simulink model "PowerFlow_SUSAN"  (R2022b)
settings: Solver=FixedStepAuto  StartTime=0.0  StopTime=10  FixedStep=0.02  RelTol=1e-3
libraries: Lib_EMTAT x193
(part 2 of 3)

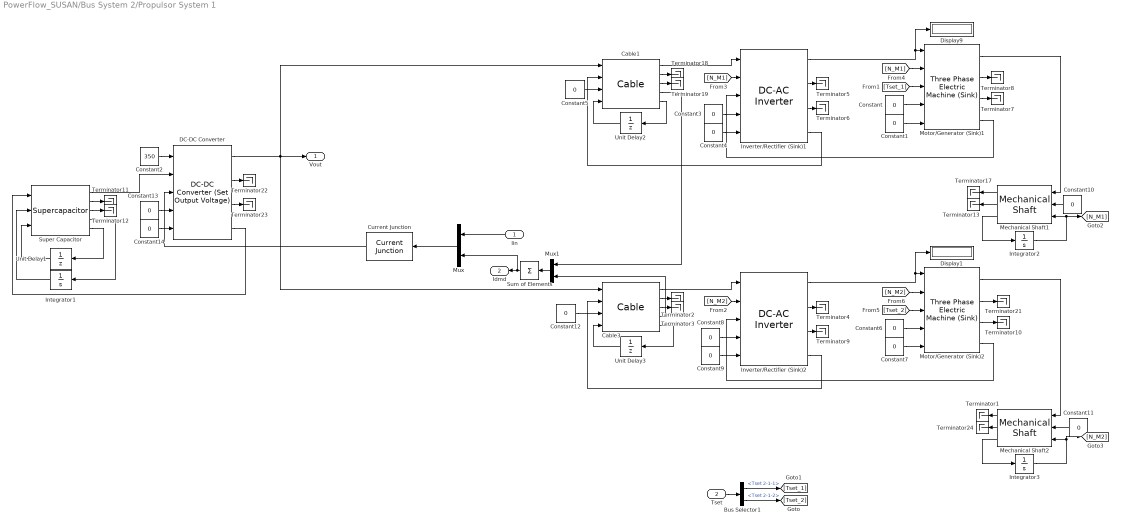
== system PowerFlow_SUSAN/Bus System 2/Propulsor System 1 ==
  Iin : Inport
  Tset : Inport  Port=2
  Bus Selector1 : BusSelector  OutputSignals=Tset 2-1-1,Tset 2-1-2
  Cable1 : Lib_EMTAT/Components/Power Flow/Cable  R=0.2
      settings: SourceProductName=EMTAT
  Cable3 : Lib_EMTAT/Components/Power Flow/Cable  R=0.2
      settings: SourceProductName=EMTAT
  Constant{,1,3..14} (14 alike) : Constant  Value=0
  Constant2 : Constant  Value=350
  Current Junction : Lib_EMTAT/Components/Power Flow/Current Junction  Nb=1
      settings: SourceProductName=EMTAT
      settings: AttributesFormatString=|
      | Current Junction
      | Version: %<LibraryVersion>
  DC-DC Converter : Lib_EMTAT/Components/Power Flow/DC-DC Converter (Set Output Voltage)  X_Vin_VoltageVec_M=[0 100 1000 5000]  Y_Iout_CurrentVec_M=[0 10 100 150]  T_C_PlossArray_M=0.98*ones(4,4)  FM=0  Plosslim=0
      settings: SourceProductName=EMTAT
  Display1 : Display
  Display9 : Display
  Integrator1 : Integrator  InitialCondition=150
  Integrator2 : Integrator  InitialCondition=2000
  Integrator3 : Integrator  InitialCondition=2000
  Inverter/Rectifier (Sink)1 : Lib_EMTAT/Components/Power Flow/DC-AC Inverter  X_C_VoltageInVec_M=[0 400]  Y_C_RMSCurrentOutVec_M=[0 300]  T_C_PowLossArray_M=[1000 1000;1000 1000]  K_e=0.0503  FM=0  Plosslim=0
      settings: SourceProductName=EMTAT
  Inverter/Rectifier (Sink)2 : Lib_EMTAT/Components/Power Flow/DC-AC Inverter  X_C_VoltageInVec_M=[0 400]  Y_C_RMSCurrentOutVec_M=[0 300]  T_C_PowLossArray_M=[1000 1000;1000 1000]  K_e=0.0503  FM=0  Plosslim=0
      settings: SourceProductName=EMTAT
  Mechanical Shaft1 : Lib_EMTAT/Components/Power Flow/Mechanical Shaft  J=0.01  B=0.001
      settings: SourceProductName=EMTAT
  Mechanical Shaft2 : Lib_EMTAT/Components/Power Flow/Mechanical Shaft  J=0.01  B=0.001
      settings: SourceProductName=EMTAT
  Motor/Generator (Sink)1 : Lib_EMTAT/Components/Power Flow/Three Phase Electric Machine (Sink)  X_C_SpeedVec_M=[0 100 1000 5000]  Y_C_TorqueVec_M=[0 10 100 150]  T_C_EffArray_M=0.99*ones(4,4)  FM=0
      settings: SourceProductName=EMTAT
  Motor/Generator (Sink)2 : Lib_EMTAT/Components/Power Flow/Three Phase Electric Machine (Sink)  X_C_SpeedVec_M=[0 100 1000 5000]  Y_C_TorqueVec_M=[0 10 100 150]  T_C_EffArray_M=0.99*ones(4,4)  FM=0
      settings: SourceProductName=EMTAT
  Mux : Mux  Inputs=2
  Mux1 : Mux  Inputs=2
  Sum of Elements : Sum  Inputs=+
  Super Capacitor : Lib_EMTAT/Components/Power Flow/Supercapacitor  C=130  ESR=0.02  TSE=0  BlkNm=double(gcb)
      settings: SourceProductName=EMTAT
  Terminator{1..13,17..19,21..24} (20 alike) : Terminator
  Unit Delay1 : UnitDelay  SampleTime=-1  HasFrameUpgradeWarning=on
  Unit Delay2 : UnitDelay  SampleTime=-1  HasFrameUpgradeWarning=on
  Unit Delay3 : UnitDelay  SampleTime=-1  HasFrameUpgradeWarning=on
  Vout : Outport
  Idmd : Outport  Port=2
  wires:
  Constant14/1 -> DC-DC Converter/5
  Constant13/1 -> DC-DC Converter/4
  Constant12/1 -> Cable3/3
  Mechanical Shaft2/2 -> Terminator24/1
  Mechanical Shaft2/1 -> Terminator1/1
  Constant11/1 -> Mechanical Shaft2/2
  Constant10/1 -> Mechanical Shaft1/2
  Mechanical Shaft1/3 -> Integrator2/1
  Motor/Generator (Sink)2/3 -> Terminator10/1
  Constant8/1 -> Inverter/Rectifier (Sink)2/4
  Inverter/Rectifier (Sink)2/1 -> Display1/1, Motor/Generator (Sink)2/1
  [N_M2] -> Motor/Generator (Sink)2/2
  Cable3/1 -> Inverter/Rectifier (Sink)2/1
  Motor/Generator (Sink)2/4 -> Inverter/Rectifier (Sink)2/3
  Constant6/1 -> Motor/Generator (Sink)2/4
  Inverter/Rectifier (Sink)2/4 -> Cable3/2
  [Tset_2] -> Motor/Generator (Sink)2/3
  Inverter/Rectifier (Sink)2/3 -> Terminator9/1
  [N_M2] -> Inverter/Rectifier (Sink)2/2
  Constant7/1 -> Motor/Generator (Sink)2/5
  Inverter/Rectifier (Sink)2/2 -> Terminator4/1
  Constant9/1 -> Inverter/Rectifier (Sink)2/5
  Constant5/1 -> Cable1/3
  Constant4/1 -> Inverter/Rectifier (Sink)1/5
  Constant3/1 -> Inverter/Rectifier (Sink)1/4
  Motor/Generator (Sink)1/3 -> Terminator7/1
  Constant1/1 -> Motor/Generator (Sink)1/5
  Constant/1 -> Motor/Generator (Sink)1/4
  Tset/1 -> Bus Selector1/1
  Bus Selector1/2 -> [Tset_2]  "<Tset 2-1-2>"
  Bus Selector1/1 -> [Tset_1]  "<Tset 2-1-1>"
  Sum of Elements/1 -> Idmd/1, Mux/2
  Mux1/1 -> Sum of Elements/1
  Motor/Generator (Sink)1/1 -> Mechanical Shaft1/1
  Inverter/Rectifier (Sink)1/2 -> Terminator5/1
  DC-DC Converter/3 -> Terminator23/1
  DC-DC Converter/2 -> Terminator22/1
  Mechanical Shaft1/1 -> Terminator17/1
  Motor/Generator (Sink)2/2 -> Terminator21/1
  Super Capacitor/3 -> Terminator12/1
  Cable1/2 -> Terminator18/1
  Motor/Generator (Sink)2/1 -> Mechanical Shaft2/1
  Cable3/3 -> Terminator3/1
  Motor/Generator (Sink)1/2 -> Terminator8/1
  Constant2/1 -> DC-DC Converter/1
  Cable1/4 -> Mux1/1
  Unit Delay1/1 -> Super Capacitor/3
  Super Capacitor/5 -> Unit Delay1/1
  Inverter/Rectifier (Sink)1/3 -> Terminator6/1
  Cable1/5 -> Unit Delay2/1
  Integrator1/1 -> Super Capacitor/2
  Inverter/Rectifier (Sink)1/4 -> Cable1/2
  Unit Delay3/1 -> Cable3/4
  Cable1/3 -> Terminator19/1
  Integrator3/1 -> Mechanical Shaft2/3, [N_M2]
  Cable3/4 -> Mux1/2
  Super Capacitor/2 -> Terminator11/1
  Inverter/Rectifier (Sink)1/1 -> Display9/1, Motor/Generator (Sink)1/1
  Cable3/5 -> Unit Delay3/1
  [N_M1] -> Inverter/Rectifier (Sink)1/2
  Cable1/1 -> Inverter/Rectifier (Sink)1/1
  Integrator2/1 -> Mechanical Shaft1/3, [N_M1]
  Mux/1 -> Current Junction/1
  Current Junction/1 -> DC-DC Converter/3
  DC-DC Converter/4 -> Super Capacitor/1
  Cable3/2 -> Terminator2/1
  Unit Delay2/1 -> Cable1/4
  Mechanical Shaft1/2 -> Terminator13/1
  [N_M1] -> Motor/Generator (Sink)1/2
  Super Capacitor/1 -> DC-DC Converter/2
  Super Capacitor/4 -> Integrator1/1
  Motor/Generator (Sink)1/4 -> Inverter/Rectifier (Sink)1/3
  DC-DC Converter/1 -> Cable1/1, Vout/1, Cable3/1
  [Tset_1] -> Motor/Generator (Sink)1/3
  Mechanical Shaft2/3 -> Integrator3/1
  Iin/1 -> Mux/1

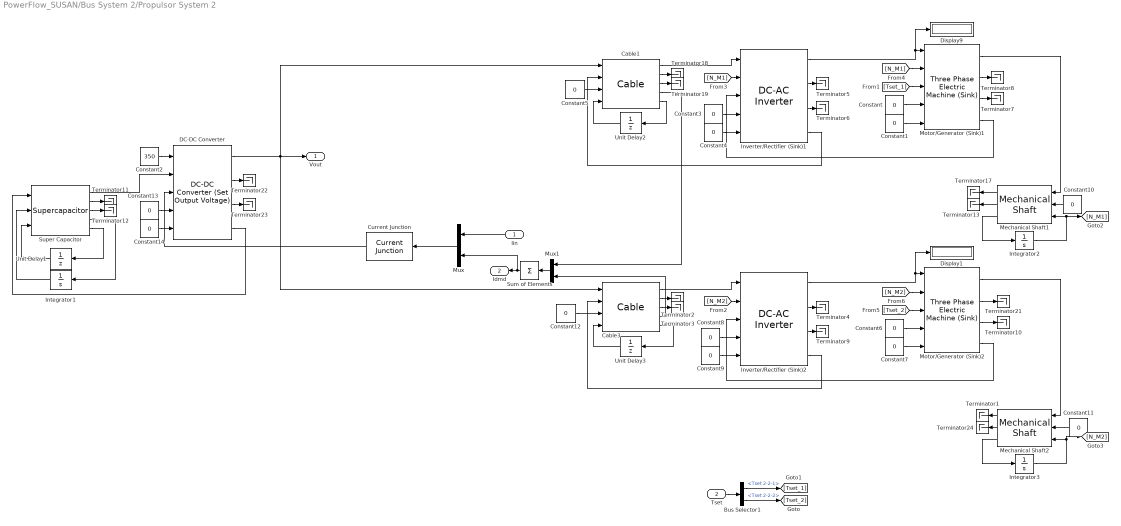
== system PowerFlow_SUSAN/Bus System 2/Propulsor System 2 ==
  Iin : Inport
  Tset : Inport  Port=2
  Bus Selector1 : BusSelector  OutputSignals=Tset 2-2-1,Tset 2-2-2
  Cable1 : Lib_EMTAT/Components/Power Flow/Cable  R=0.2
      settings: SourceProductName=EMTAT
  Cable3 : Lib_EMTAT/Components/Power Flow/Cable  R=0.2
      settings: SourceProductName=EMTAT
  Constant{,1,3..14} (14 alike) : Constant  Value=0
  Constant2 : Constant  Value=350
  Current Junction : Lib_EMTAT/Components/Power Flow/Current Junction  Nb=1
      settings: SourceProductName=EMTAT
      settings: AttributesFormatString=|
      | Current Junction
      | Version: %<LibraryVersion>
  DC-DC Converter : Lib_EMTAT/Components/Power Flow/DC-DC Converter (Set Output Voltage)  X_Vin_VoltageVec_M=[0 100 1000 5000]  Y_Iout_CurrentVec_M=[0 10 100 150]  T_C_PlossArray_M=0.98*ones(4,4)  FM=0  Plosslim=0
      settings: SourceProductName=EMTAT
  Display1 : Display
  Display9 : Display
  Integrator1 : Integrator  InitialCondition=150
  Integrator2 : Integrator  InitialCondition=2000
  Integrator3 : Integrator  InitialCondition=2000
  Inverter/Rectifier (Sink)1 : Lib_EMTAT/Components/Power Flow/DC-AC Inverter  X_C_VoltageInVec_M=[0 400]  Y_C_RMSCurrentOutVec_M=[0 300]  T_C_PowLossArray_M=[1000 1000;1000 1000]  K_e=0.0503  FM=0  Plosslim=0
      settings: SourceProductName=EMTAT
  Inverter/Rectifier (Sink)2 : Lib_EMTAT/Components/Power Flow/DC-AC Inverter  X_C_VoltageInVec_M=[0 400]  Y_C_RMSCurrentOutVec_M=[0 300]  T_C_PowLossArray_M=[1000 1000;1000 1000]  K_e=0.0503  FM=0  Plosslim=0
      settings: SourceProductName=EMTAT
  Mechanical Shaft1 : Lib_EMTAT/Components/Power Flow/Mechanical Shaft  J=0.01  B=0.001
      settings: SourceProductName=EMTAT
  Mechanical Shaft2 : Lib_EMTAT/Components/Power Flow/Mechanical Shaft  J=0.01  B=0.001
      settings: SourceProductName=EMTAT
  Motor/Generator (Sink)1 : Lib_EMTAT/Components/Power Flow/Three Phase Electric Machine (Sink)  X_C_SpeedVec_M=[0 100 1000 5000]  Y_C_TorqueVec_M=[0 10 100 150]  T_C_EffArray_M=0.99*ones(4,4)  FM=0
      settings: SourceProductName=EMTAT
  Motor/Generator (Sink)2 : Lib_EMTAT/Components/Power Flow/Three Phase Electric Machine (Sink)  X_C_SpeedVec_M=[0 100 1000 5000]  Y_C_TorqueVec_M=[0 10 100 150]  T_C_EffArray_M=0.99*ones(4,4)  FM=0
      settings: SourceProductName=EMTAT
  Mux : Mux  Inputs=2
  Mux1 : Mux  Inputs=2
  Sum of Elements : Sum  Inputs=+
  Super Capacitor : Lib_EMTAT/Components/Power Flow/Supercapacitor  C=130  ESR=0.02  TSE=0  BlkNm=double(gcb)
      settings: SourceProductName=EMTAT
  Terminator{1..13,17..19,21..24} (20 alike) : Terminator
  Unit Delay1 : UnitDelay  SampleTime=-1  HasFrameUpgradeWarning=on
  Unit Delay2 : UnitDelay  SampleTime=-1  HasFrameUpgradeWarning=on
  Unit Delay3 : UnitDelay  SampleTime=-1  HasFrameUpgradeWarning=on
  Vout : Outport
  Idmd : Outport  Port=2
  wires:
  Iin/1 -> Mux/1
  Mechanical Shaft2/3 -> Integrator3/1
  [Tset_1] -> Motor/Generator (Sink)1/3
  DC-DC Converter/1 -> Cable3/1, Vout/1, Cable1/1
  Motor/Generator (Sink)1/4 -> Inverter/Rectifier (Sink)1/3
  Super Capacitor/4 -> Integrator1/1
  Super Capacitor/1 -> DC-DC Converter/2
  [N_M1] -> Motor/Generator (Sink)1/2
  Mechanical Shaft1/2 -> Terminator13/1
  Unit Delay2/1 -> Cable1/4
  Cable3/2 -> Terminator2/1
  DC-DC Converter/4 -> Super Capacitor/1
  Current Junction/1 -> DC-DC Converter/3
  Mux/1 -> Current Junction/1
  Integrator2/1 -> [N_M1], Mechanical Shaft1/3
  Cable1/1 -> Inverter/Rectifier (Sink)1/1
  [N_M1] -> Inverter/Rectifier (Sink)1/2
  Cable3/5 -> Unit Delay3/1
  Inverter/Rectifier (Sink)1/1 -> Motor/Generator (Sink)1/1, Display9/1
  Super Capacitor/2 -> Terminator11/1
  Cable3/4 -> Mux1/2
  Integrator3/1 -> [N_M2], Mechanical Shaft2/3
  Cable1/3 -> Terminator19/1
  Unit Delay3/1 -> Cable3/4
  Inverter/Rectifier (Sink)1/4 -> Cable1/2
  Integrator1/1 -> Super Capacitor/2
  Cable1/5 -> Unit Delay2/1
  Inverter/Rectifier (Sink)1/3 -> Terminator6/1
  Super Capacitor/5 -> Unit Delay1/1
  Unit Delay1/1 -> Super Capacitor/3
  Cable1/4 -> Mux1/1
  Constant2/1 -> DC-DC Converter/1
  Motor/Generator (Sink)1/2 -> Terminator8/1
  Cable3/3 -> Terminator3/1
  Motor/Generator (Sink)2/1 -> Mechanical Shaft2/1
  Cable1/2 -> Terminator18/1
  Super Capacitor/3 -> Terminator12/1
  Motor/Generator (Sink)2/2 -> Terminator21/1
  Mechanical Shaft1/1 -> Terminator17/1
  DC-DC Converter/2 -> Terminator22/1
  DC-DC Converter/3 -> Terminator23/1
  Inverter/Rectifier (Sink)1/2 -> Terminator5/1
  Motor/Generator (Sink)1/1 -> Mechanical Shaft1/1
  Mux1/1 -> Sum of Elements/1
  Sum of Elements/1 -> Mux/2, Idmd/1
  Bus Selector1/1 -> [Tset_1]  "<Tset 2-2-1>"
  Bus Selector1/2 -> [Tset_2]  "<Tset 2-2-2>"
  Tset/1 -> Bus Selector1/1
  Constant/1 -> Motor/Generator (Sink)1/4
  Constant1/1 -> Motor/Generator (Sink)1/5
  Motor/Generator (Sink)1/3 -> Terminator7/1
  Constant3/1 -> Inverter/Rectifier (Sink)1/4
  Constant4/1 -> Inverter/Rectifier (Sink)1/5
  Constant5/1 -> Cable1/3
  Constant9/1 -> Inverter/Rectifier (Sink)2/5
  Inverter/Rectifier (Sink)2/2 -> Terminator4/1
  Constant7/1 -> Motor/Generator (Sink)2/5
  [N_M2] -> Inverter/Rectifier (Sink)2/2
  Inverter/Rectifier (Sink)2/3 -> Terminator9/1
  [Tset_2] -> Motor/Generator (Sink)2/3
  Inverter/Rectifier (Sink)2/4 -> Cable3/2
  Constant6/1 -> Motor/Generator (Sink)2/4
  Motor/Generator (Sink)2/4 -> Inverter/Rectifier (Sink)2/3
  Cable3/1 -> Inverter/Rectifier (Sink)2/1
  [N_M2] -> Motor/Generator (Sink)2/2
  Inverter/Rectifier (Sink)2/1 -> Motor/Generator (Sink)2/1, Display1/1
  Constant8/1 -> Inverter/Rectifier (Sink)2/4
  Motor/Generator (Sink)2/3 -> Terminator10/1
  Mechanical Shaft1/3 -> Integrator2/1
  Constant10/1 -> Mechanical Shaft1/2
  Constant11/1 -> Mechanical Shaft2/2
  Mechanical Shaft2/1 -> Terminator1/1
  Mechanical Shaft2/2 -> Terminator24/1
  Constant12/1 -> Cable3/3
  Constant13/1 -> DC-DC Converter/4
  Constant14/1 -> DC-DC Converter/5

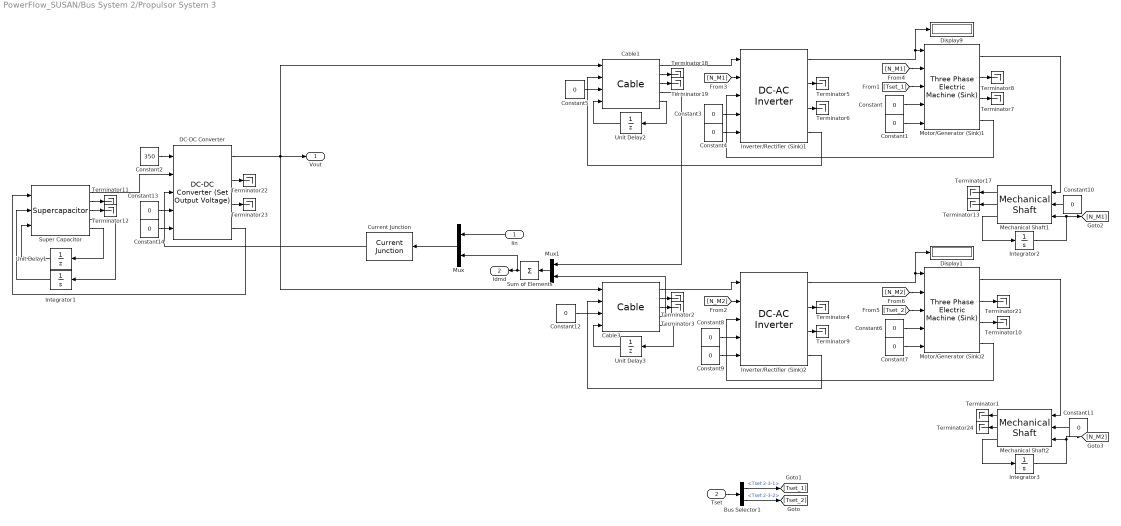
== system PowerFlow_SUSAN/Bus System 2/Propulsor System 3 ==
  Iin : Inport
  Tset : Inport  Port=2
  Bus Selector1 : BusSelector  OutputSignals=Tset 2-3-1,Tset 2-3-2
  Cable1 : Lib_EMTAT/Components/Power Flow/Cable  R=0.2
      settings: SourceProductName=EMTAT
  Cable3 : Lib_EMTAT/Components/Power Flow/Cable  R=0.2
      settings: SourceProductName=EMTAT
  Constant{,1,3..14} (14 alike) : Constant  Value=0
  Constant2 : Constant  Value=350
  Current Junction : Lib_EMTAT/Components/Power Flow/Current Junction  Nb=1
      settings: SourceProductName=EMTAT
      settings: AttributesFormatString=|
      | Current Junction
      | Version: %<LibraryVersion>
  DC-DC Converter : Lib_EMTAT/Components/Power Flow/DC-DC Converter (Set Output Voltage)  X_Vin_VoltageVec_M=[0 100 1000 5000]  Y_Iout_CurrentVec_M=[0 10 100 150]  T_C_PlossArray_M=0.98*ones(4,4)  FM=0  Plosslim=0
      settings: SourceProductName=EMTAT
  Display1 : Display
  Display9 : Display
  Integrator1 : Integrator  InitialCondition=150
  Integrator2 : Integrator  InitialCondition=2000
  Integrator3 : Integrator  InitialCondition=2000
  Inverter/Rectifier (Sink)1 : Lib_EMTAT/Components/Power Flow/DC-AC Inverter  X_C_VoltageInVec_M=[0 400]  Y_C_RMSCurrentOutVec_M=[0 300]  T_C_PowLossArray_M=[1000 1000;1000 1000]  K_e=0.0503  FM=0  Plosslim=0
      settings: SourceProductName=EMTAT
  Inverter/Rectifier (Sink)2 : Lib_EMTAT/Components/Power Flow/DC-AC Inverter  X_C_VoltageInVec_M=[0 400]  Y_C_RMSCurrentOutVec_M=[0 300]  T_C_PowLossArray_M=[1000 1000;1000 1000]  K_e=0.0503  FM=0  Plosslim=0
      settings: SourceProductName=EMTAT
  Mechanical Shaft1 : Lib_EMTAT/Components/Power Flow/Mechanical Shaft  J=0.01  B=0.001
      settings: SourceProductName=EMTAT
  Mechanical Shaft2 : Lib_EMTAT/Components/Power Flow/Mechanical Shaft  J=0.01  B=0.001
      settings: SourceProductName=EMTAT
  Motor/Generator (Sink)1 : Lib_EMTAT/Components/Power Flow/Three Phase Electric Machine (Sink)  X_C_SpeedVec_M=[0 100 1000 5000]  Y_C_TorqueVec_M=[0 10 100 150]  T_C_EffArray_M=0.99*ones(4,4)  FM=0
      settings: SourceProductName=EMTAT
  Motor/Generator (Sink)2 : Lib_EMTAT/Components/Power Flow/Three Phase Electric Machine (Sink)  X_C_SpeedVec_M=[0 100 1000 5000]  Y_C_TorqueVec_M=[0 10 100 150]  T_C_EffArray_M=0.99*ones(4,4)  FM=0
      settings: SourceProductName=EMTAT
  Mux : Mux  Inputs=2
  Mux1 : Mux  Inputs=2
  Sum of Elements : Sum  Inputs=+
  Super Capacitor : Lib_EMTAT/Components/Power Flow/Supercapacitor  C=130  ESR=0.02  TSE=0  BlkNm=double(gcb)
      settings: SourceProductName=EMTAT
  Terminator{1..13,17..19,21..24} (20 alike) : Terminator
  Unit Delay1 : UnitDelay  SampleTime=-1  HasFrameUpgradeWarning=on
  Unit Delay2 : UnitDelay  SampleTime=-1  HasFrameUpgradeWarning=on
  Unit Delay3 : UnitDelay  SampleTime=-1  HasFrameUpgradeWarning=on
  Vout : Outport
  Idmd : Outport  Port=2
  wires:
  Constant14/1 -> DC-DC Converter/5
  Constant13/1 -> DC-DC Converter/4
  Constant12/1 -> Cable3/3
  Mechanical Shaft2/2 -> Terminator24/1
  Mechanical Shaft2/1 -> Terminator1/1
  Constant11/1 -> Mechanical Shaft2/2
  Constant10/1 -> Mechanical Shaft1/2
  Mechanical Shaft1/3 -> Integrator2/1
  Motor/Generator (Sink)2/3 -> Terminator10/1
  Constant8/1 -> Inverter/Rectifier (Sink)2/4
  Inverter/Rectifier (Sink)2/1 -> Display1/1, Motor/Generator (Sink)2/1
  [N_M2] -> Motor/Generator (Sink)2/2
  Cable3/1 -> Inverter/Rectifier (Sink)2/1
  Motor/Generator (Sink)2/4 -> Inverter/Rectifier (Sink)2/3
  Constant6/1 -> Motor/Generator (Sink)2/4
  Inverter/Rectifier (Sink)2/4 -> Cable3/2
  [Tset_2] -> Motor/Generator (Sink)2/3
  Inverter/Rectifier (Sink)2/3 -> Terminator9/1
  [N_M2] -> Inverter/Rectifier (Sink)2/2
  Constant7/1 -> Motor/Generator (Sink)2/5
  Inverter/Rectifier (Sink)2/2 -> Terminator4/1
  Constant9/1 -> Inverter/Rectifier (Sink)2/5
  Constant5/1 -> Cable1/3
  Constant4/1 -> Inverter/Rectifier (Sink)1/5
  Constant3/1 -> Inverter/Rectifier (Sink)1/4
  Motor/Generator (Sink)1/3 -> Terminator7/1
  Constant1/1 -> Motor/Generator (Sink)1/5
  Constant/1 -> Motor/Generator (Sink)1/4
  Tset/1 -> Bus Selector1/1
  Bus Selector1/2 -> [Tset_2]  "<Tset 2-3-2>"
  Bus Selector1/1 -> [Tset_1]  "<Tset 2-3-1>"
  Sum of Elements/1 -> Idmd/1, Mux/2
  Mux1/1 -> Sum of Elements/1
  Motor/Generator (Sink)1/1 -> Mechanical Shaft1/1
  Inverter/Rectifier (Sink)1/2 -> Terminator5/1
  DC-DC Converter/3 -> Terminator23/1
  DC-DC Converter/2 -> Terminator22/1
  Mechanical Shaft1/1 -> Terminator17/1
  Motor/Generator (Sink)2/2 -> Terminator21/1
  Super Capacitor/3 -> Terminator12/1
  Cable1/2 -> Terminator18/1
  Motor/Generator (Sink)2/1 -> Mechanical Shaft2/1
  Cable3/3 -> Terminator3/1
  Motor/Generator (Sink)1/2 -> Terminator8/1
  Constant2/1 -> DC-DC Converter/1
  Cable1/4 -> Mux1/1
  Unit Delay1/1 -> Super Capacitor/3
  Super Capacitor/5 -> Unit Delay1/1
  Inverter/Rectifier (Sink)1/3 -> Terminator6/1
  Cable1/5 -> Unit Delay2/1
  Integrator1/1 -> Super Capacitor/2
  Inverter/Rectifier (Sink)1/4 -> Cable1/2
  Unit Delay3/1 -> Cable3/4
  Cable1/3 -> Terminator19/1
  Integrator3/1 -> Mechanical Shaft2/3, [N_M2]
  Cable3/4 -> Mux1/2
  Super Capacitor/2 -> Terminator11/1
  Inverter/Rectifier (Sink)1/1 -> Display9/1, Motor/Generator (Sink)1/1
  Cable3/5 -> Unit Delay3/1
  [N_M1] -> Inverter/Rectifier (Sink)1/2
  Cable1/1 -> Inverter/Rectifier (Sink)1/1
  Integrator2/1 -> Mechanical Shaft1/3, [N_M1]
  Mux/1 -> Current Junction/1
  Current Junction/1 -> DC-DC Converter/3
  DC-DC Converter/4 -> Super Capacitor/1
  Cable3/2 -> Terminator2/1
  Unit Delay2/1 -> Cable1/4
  Mechanical Shaft1/2 -> Terminator13/1
  [N_M1] -> Motor/Generator (Sink)1/2
  Super Capacitor/1 -> DC-DC Converter/2
  Super Capacitor/4 -> Integrator1/1
  Motor/Generator (Sink)1/4 -> Inverter/Rectifier (Sink)1/3
  DC-DC Converter/1 -> Cable1/1, Vout/1, Cable3/1
  [Tset_1] -> Motor/Generator (Sink)1/3
  Mechanical Shaft2/3 -> Integrator3/1
  Iin/1 -> Mux/1

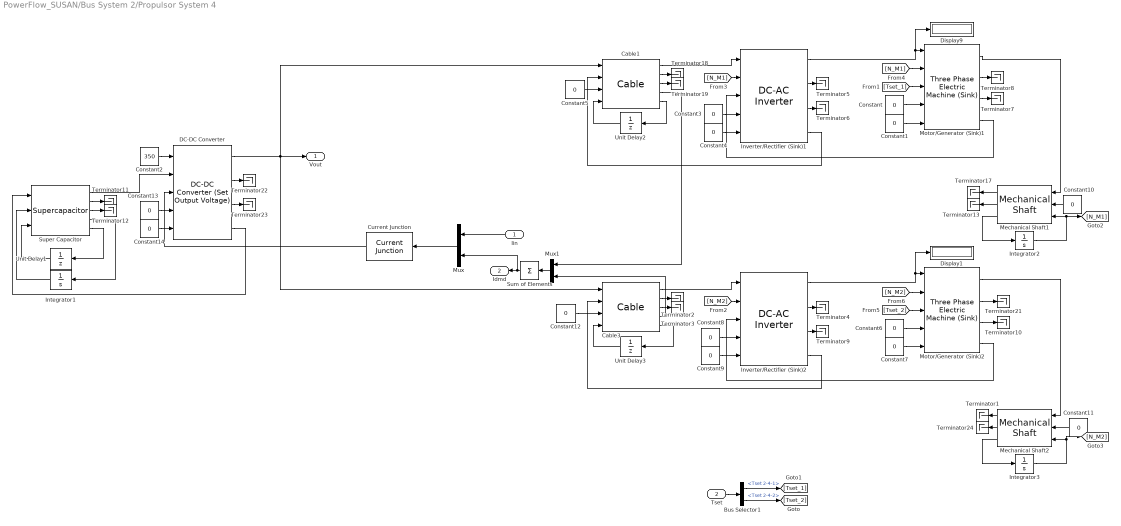
== system PowerFlow_SUSAN/Bus System 2/Propulsor System 4 ==
  Iin : Inport
  Tset : Inport  Port=2
  Bus Selector1 : BusSelector  OutputSignals=Tset 2-4-1,Tset 2-4-2
  Cable1 : Lib_EMTAT/Components/Power Flow/Cable  R=0.2
      settings: SourceProductName=EMTAT
  Cable3 : Lib_EMTAT/Components/Power Flow/Cable  R=0.2
      settings: SourceProductName=EMTAT
  Constant{,1,3..14} (14 alike) : Constant  Value=0
  Constant2 : Constant  Value=350
  Current Junction : Lib_EMTAT/Components/Power Flow/Current Junction  Nb=1
      settings: SourceProductName=EMTAT
      settings: AttributesFormatString=|
      | Current Junction
      | Version: %<LibraryVersion>
  DC-DC Converter : Lib_EMTAT/Components/Power Flow/DC-DC Converter (Set Output Voltage)  X_Vin_VoltageVec_M=[0 100 1000 5000]  Y_Iout_CurrentVec_M=[0 10 100 150]  T_C_PlossArray_M=0.98*ones(4,4)  FM=0  Plosslim=0
      settings: SourceProductName=EMTAT
  Display1 : Display
  Display9 : Display
  Integrator1 : Integrator  InitialCondition=150
  Integrator2 : Integrator  InitialCondition=2000
  Integrator3 : Integrator  InitialCondition=2000
  Inverter/Rectifier (Sink)1 : Lib_EMTAT/Components/Power Flow/DC-AC Inverter  X_C_VoltageInVec_M=[0 400]  Y_C_RMSCurrentOutVec_M=[0 300]  T_C_PowLossArray_M=[1000 1000;1000 1000]  K_e=0.0503  FM=0  Plosslim=0
      settings: SourceProductName=EMTAT
  Inverter/Rectifier (Sink)2 : Lib_EMTAT/Components/Power Flow/DC-AC Inverter  X_C_VoltageInVec_M=[0 400]  Y_C_RMSCurrentOutVec_M=[0 300]  T_C_PowLossArray_M=[1000 1000;1000 1000]  K_e=0.0503  FM=0  Plosslim=0
      settings: SourceProductName=EMTAT
  Mechanical Shaft1 : Lib_EMTAT/Components/Power Flow/Mechanical Shaft  J=0.01  B=0.001
      settings: SourceProductName=EMTAT
  Mechanical Shaft2 : Lib_EMTAT/Components/Power Flow/Mechanical Shaft  J=0.01  B=0.001
      settings: SourceProductName=EMTAT
  Motor/Generator (Sink)1 : Lib_EMTAT/Components/Power Flow/Three Phase Electric Machine (Sink)  X_C_SpeedVec_M=[0 100 1000 5000]  Y_C_TorqueVec_M=[0 10 100 150]  T_C_EffArray_M=0.99*ones(4,4)  FM=0
      settings: SourceProductName=EMTAT
  Motor/Generator (Sink)2 : Lib_EMTAT/Components/Power Flow/Three Phase Electric Machine (Sink)  X_C_SpeedVec_M=[0 100 1000 5000]  Y_C_TorqueVec_M=[0 10 100 150]  T_C_EffArray_M=0.99*ones(4,4)  FM=0
      settings: SourceProductName=EMTAT
  Mux : Mux  Inputs=2
  Mux1 : Mux  Inputs=2
  Sum of Elements : Sum  Inputs=+
  Super Capacitor : Lib_EMTAT/Components/Power Flow/Supercapacitor  C=130  ESR=0.02  TSE=0  BlkNm=double(gcb)
      settings: SourceProductName=EMTAT
  Terminator{1..13,17..19,21..24} (20 alike) : Terminator
  Unit Delay1 : UnitDelay  SampleTime=-1  HasFrameUpgradeWarning=on
  Unit Delay2 : UnitDelay  SampleTime=-1  HasFrameUpgradeWarning=on
  Unit Delay3 : UnitDelay  SampleTime=-1  HasFrameUpgradeWarning=on
  Vout : Outport
  Idmd : Outport  Port=2
  wires:
  Iin/1 -> Mux/1
  Mechanical Shaft2/3 -> Integrator3/1
  [Tset_1] -> Motor/Generator (Sink)1/3
  DC-DC Converter/1 -> Cable3/1, Vout/1, Cable1/1
  Motor/Generator (Sink)1/4 -> Inverter/Rectifier (Sink)1/3
  Super Capacitor/4 -> Integrator1/1
  Super Capacitor/1 -> DC-DC Converter/2
  [N_M1] -> Motor/Generator (Sink)1/2
  Mechanical Shaft1/2 -> Terminator13/1
  Unit Delay2/1 -> Cable1/4
  Cable3/2 -> Terminator2/1
  DC-DC Converter/4 -> Super Capacitor/1
  Current Junction/1 -> DC-DC Converter/3
  Mux/1 -> Current Junction/1
  Integrator2/1 -> [N_M1], Mechanical Shaft1/3
  Cable1/1 -> Inverter/Rectifier (Sink)1/1
  [N_M1] -> Inverter/Rectifier (Sink)1/2
  Cable3/5 -> Unit Delay3/1
  Inverter/Rectifier (Sink)1/1 -> Motor/Generator (Sink)1/1, Display9/1
  Super Capacitor/2 -> Terminator11/1
  Cable3/4 -> Mux1/2
  Integrator3/1 -> [N_M2], Mechanical Shaft2/3
  Cable1/3 -> Terminator19/1
  Unit Delay3/1 -> Cable3/4
  Inverter/Rectifier (Sink)1/4 -> Cable1/2
  Integrator1/1 -> Super Capacitor/2
  Cable1/5 -> Unit Delay2/1
  Inverter/Rectifier (Sink)1/3 -> Terminator6/1
  Super Capacitor/5 -> Unit Delay1/1
  Unit Delay1/1 -> Super Capacitor/3
  Cable1/4 -> Mux1/1
  Constant2/1 -> DC-DC Converter/1
  Motor/Generator (Sink)1/2 -> Terminator8/1
  Cable3/3 -> Terminator3/1
  Motor/Generator (Sink)2/1 -> Mechanical Shaft2/1
  Cable1/2 -> Terminator18/1
  Super Capacitor/3 -> Terminator12/1
  Motor/Generator (Sink)2/2 -> Terminator21/1
  Mechanical Shaft1/1 -> Terminator17/1
  DC-DC Converter/2 -> Terminator22/1
  DC-DC Converter/3 -> Terminator23/1
  Inverter/Rectifier (Sink)1/2 -> Terminator5/1
  Motor/Generator (Sink)1/1 -> Mechanical Shaft1/1
  Mux1/1 -> Sum of Elements/1
  Sum of Elements/1 -> Mux/2, Idmd/1
  Bus Selector1/1 -> [Tset_1]  "<Tset 2-4-1>"
  Bus Selector1/2 -> [Tset_2]  "<Tset 2-4-2>"
  Tset/1 -> Bus Selector1/1
  Constant/1 -> Motor/Generator (Sink)1/4
  Constant1/1 -> Motor/Generator (Sink)1/5
  Motor/Generator (Sink)1/3 -> Terminator7/1
  Constant3/1 -> Inverter/Rectifier (Sink)1/4
  Constant4/1 -> Inverter/Rectifier (Sink)1/5
  Constant5/1 -> Cable1/3
  Constant9/1 -> Inverter/Rectifier (Sink)2/5
  Inverter/Rectifier (Sink)2/2 -> Terminator4/1
  Constant7/1 -> Motor/Generator (Sink)2/5
  [N_M2] -> Inverter/Rectifier (Sink)2/2
  Inverter/Rectifier (Sink)2/3 -> Terminator9/1
  [Tset_2] -> Motor/Generator (Sink)2/3
  Inverter/Rectifier (Sink)2/4 -> Cable3/2
  Constant6/1 -> Motor/Generator (Sink)2/4
  Motor/Generator (Sink)2/4 -> Inverter/Rectifier (Sink)2/3
  Cable3/1 -> Inverter/Rectifier (Sink)2/1
  [N_M2] -> Motor/Generator (Sink)2/2
  Inverter/Rectifier (Sink)2/1 -> Motor/Generator (Sink)2/1, Display1/1
  Constant8/1 -> Inverter/Rectifier (Sink)2/4
  Motor/Generator (Sink)2/3 -> Terminator10/1
  Mechanical Shaft1/3 -> Integrator2/1
  Constant10/1 -> Mechanical Shaft1/2
  Constant11/1 -> Mechanical Shaft2/2
  Mechanical Shaft2/1 -> Terminator1/1
  Mechanical Shaft2/2 -> Terminator24/1
  Constant12/1 -> Cable3/3
  Constant13/1 -> DC-DC Converter/4
  Constant14/1 -> DC-DC Converter/5

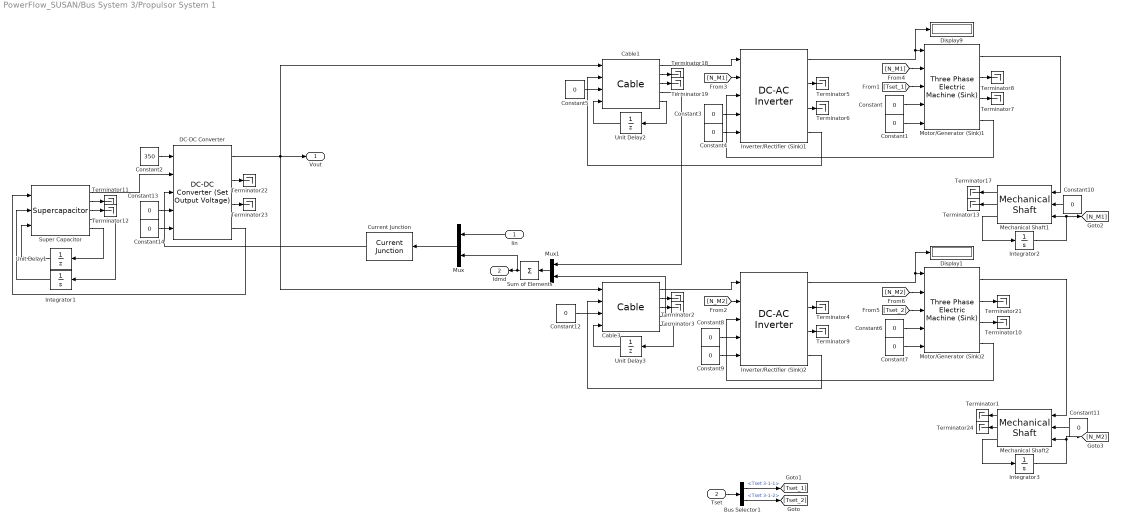
== system PowerFlow_SUSAN/Bus System 3/Propulsor System 1 ==
  Iin : Inport
  Tset : Inport  Port=2
  Bus Selector1 : BusSelector  OutputSignals=Tset 3-1-1,Tset 3-1-2
  Cable1 : Lib_EMTAT/Components/Power Flow/Cable  R=0.2
      settings: SourceProductName=EMTAT
  Cable3 : Lib_EMTAT/Components/Power Flow/Cable  R=0.2
      settings: SourceProductName=EMTAT
  Constant{,1,3..14} (14 alike) : Constant  Value=0
  Constant2 : Constant  Value=350
  Current Junction : Lib_EMTAT/Components/Power Flow/Current Junction  Nb=1
      settings: SourceProductName=EMTAT
      settings: AttributesFormatString=|
      | Current Junction
      | Version: %<LibraryVersion>
  DC-DC Converter : Lib_EMTAT/Components/Power Flow/DC-DC Converter (Set Output Voltage)  X_Vin_VoltageVec_M=[0 100 1000 5000]  Y_Iout_CurrentVec_M=[0 10 100 150]  T_C_PlossArray_M=0.98*ones(4,4)  FM=0  Plosslim=0
      settings: SourceProductName=EMTAT
  Display1 : Display
  Display9 : Display
  Integrator1 : Integrator  InitialCondition=150
  Integrator2 : Integrator  InitialCondition=2000
  Integrator3 : Integrator  InitialCondition=2000
  Inverter/Rectifier (Sink)1 : Lib_EMTAT/Components/Power Flow/DC-AC Inverter  X_C_VoltageInVec_M=[0 400]  Y_C_RMSCurrentOutVec_M=[0 300]  T_C_PowLossArray_M=[1000 1000;1000 1000]  K_e=0.0503  FM=0  Plosslim=0
      settings: SourceProductName=EMTAT
  Inverter/Rectifier (Sink)2 : Lib_EMTAT/Components/Power Flow/DC-AC Inverter  X_C_VoltageInVec_M=[0 400]  Y_C_RMSCurrentOutVec_M=[0 300]  T_C_PowLossArray_M=[1000 1000;1000 1000]  K_e=0.0503  FM=0  Plosslim=0
      settings: SourceProductName=EMTAT
  Mechanical Shaft1 : Lib_EMTAT/Components/Power Flow/Mechanical Shaft  J=0.01  B=0.001
      settings: SourceProductName=EMTAT
  Mechanical Shaft2 : Lib_EMTAT/Components/Power Flow/Mechanical Shaft  J=0.01  B=0.001
      settings: SourceProductName=EMTAT
  Motor/Generator (Sink)1 : Lib_EMTAT/Components/Power Flow/Three Phase Electric Machine (Sink)  X_C_SpeedVec_M=[0 100 1000 5000]  Y_C_TorqueVec_M=[0 10 100 150]  T_C_EffArray_M=0.99*ones(4,4)  FM=0
      settings: SourceProductName=EMTAT
  Motor/Generator (Sink)2 : Lib_EMTAT/Components/Power Flow/Three Phase Electric Machine (Sink)  X_C_SpeedVec_M=[0 100 1000 5000]  Y_C_TorqueVec_M=[0 10 100 150]  T_C_EffArray_M=0.99*ones(4,4)  FM=0
      settings: SourceProductName=EMTAT
  Mux : Mux  Inputs=2
  Mux1 : Mux  Inputs=2
  Sum of Elements : Sum  Inputs=+
  Super Capacitor : Lib_EMTAT/Components/Power Flow/Supercapacitor  C=130  ESR=0.02  TSE=0  BlkNm=double(gcb)
      settings: SourceProductName=EMTAT
  Terminator{1..13,17..19,21..24} (20 alike) : Terminator
  Unit Delay1 : UnitDelay  SampleTime=-1  HasFrameUpgradeWarning=on
  Unit Delay2 : UnitDelay  SampleTime=-1  HasFrameUpgradeWarning=on
  Unit Delay3 : UnitDelay  SampleTime=-1  HasFrameUpgradeWarning=on
  Vout : Outport
  Idmd : Outport  Port=2
  wires:
  Iin/1 -> Mux/1
  Mechanical Shaft2/3 -> Integrator3/1
  [Tset_1] -> Motor/Generator (Sink)1/3
  DC-DC Converter/1 -> Cable3/1, Vout/1, Cable1/1
  Motor/Generator (Sink)1/4 -> Inverter/Rectifier (Sink)1/3
  Super Capacitor/4 -> Integrator1/1
  Super Capacitor/1 -> DC-DC Converter/2
  [N_M1] -> Motor/Generator (Sink)1/2
  Mechanical Shaft1/2 -> Terminator13/1
  Unit Delay2/1 -> Cable1/4
  Cable3/2 -> Terminator2/1
  DC-DC Converter/4 -> Super Capacitor/1
  Current Junction/1 -> DC-DC Converter/3
  Mux/1 -> Current Junction/1
  Integrator2/1 -> [N_M1], Mechanical Shaft1/3
  Cable1/1 -> Inverter/Rectifier (Sink)1/1
  [N_M1] -> Inverter/Rectifier (Sink)1/2
  Cable3/5 -> Unit Delay3/1
  Inverter/Rectifier (Sink)1/1 -> Motor/Generator (Sink)1/1, Display9/1
  Super Capacitor/2 -> Terminator11/1
  Cable3/4 -> Mux1/2
  Integrator3/1 -> [N_M2], Mechanical Shaft2/3
  Cable1/3 -> Terminator19/1
  Unit Delay3/1 -> Cable3/4
  Inverter/Rectifier (Sink)1/4 -> Cable1/2
  Integrator1/1 -> Super Capacitor/2
  Cable1/5 -> Unit Delay2/1
  Inverter/Rectifier (Sink)1/3 -> Terminator6/1
  Super Capacitor/5 -> Unit Delay1/1
  Unit Delay1/1 -> Super Capacitor/3
  Cable1/4 -> Mux1/1
  Constant2/1 -> DC-DC Converter/1
  Motor/Generator (Sink)1/2 -> Terminator8/1
  Cable3/3 -> Terminator3/1
  Motor/Generator (Sink)2/1 -> Mechanical Shaft2/1
  Cable1/2 -> Terminator18/1
  Super Capacitor/3 -> Terminator12/1
  Motor/Generator (Sink)2/2 -> Terminator21/1
  Mechanical Shaft1/1 -> Terminator17/1
  DC-DC Converter/2 -> Terminator22/1
  DC-DC Converter/3 -> Terminator23/1
  Inverter/Rectifier (Sink)1/2 -> Terminator5/1
  Motor/Generator (Sink)1/1 -> Mechanical Shaft1/1
  Mux1/1 -> Sum of Elements/1
  Sum of Elements/1 -> Mux/2, Idmd/1
  Bus Selector1/1 -> [Tset_1]  "<Tset 3-1-1>"
  Bus Selector1/2 -> [Tset_2]  "<Tset 3-1-2>"
  Tset/1 -> Bus Selector1/1
  Constant/1 -> Motor/Generator (Sink)1/4
  Constant1/1 -> Motor/Generator (Sink)1/5
  Motor/Generator (Sink)1/3 -> Terminator7/1
  Constant3/1 -> Inverter/Rectifier (Sink)1/4
  Constant4/1 -> Inverter/Rectifier (Sink)1/5
  Constant5/1 -> Cable1/3
  Constant9/1 -> Inverter/Rectifier (Sink)2/5
  Inverter/Rectifier (Sink)2/2 -> Terminator4/1
  Constant7/1 -> Motor/Generator (Sink)2/5
  [N_M2] -> Inverter/Rectifier (Sink)2/2
  Inverter/Rectifier (Sink)2/3 -> Terminator9/1
  [Tset_2] -> Motor/Generator (Sink)2/3
  Inverter/Rectifier (Sink)2/4 -> Cable3/2
  Constant6/1 -> Motor/Generator (Sink)2/4
  Motor/Generator (Sink)2/4 -> Inverter/Rectifier (Sink)2/3
  Cable3/1 -> Inverter/Rectifier (Sink)2/1
  [N_M2] -> Motor/Generator (Sink)2/2
  Inverter/Rectifier (Sink)2/1 -> Motor/Generator (Sink)2/1, Display1/1
  Constant8/1 -> Inverter/Rectifier (Sink)2/4
  Motor/Generator (Sink)2/3 -> Terminator10/1
  Mechanical Shaft1/3 -> Integrator2/1
  Constant10/1 -> Mechanical Shaft1/2
  Constant11/1 -> Mechanical Shaft2/2
  Mechanical Shaft2/1 -> Terminator1/1
  Mechanical Shaft2/2 -> Terminator24/1
  Constant12/1 -> Cable3/3
  Constant13/1 -> DC-DC Converter/4
  Constant14/1 -> DC-DC Converter/5

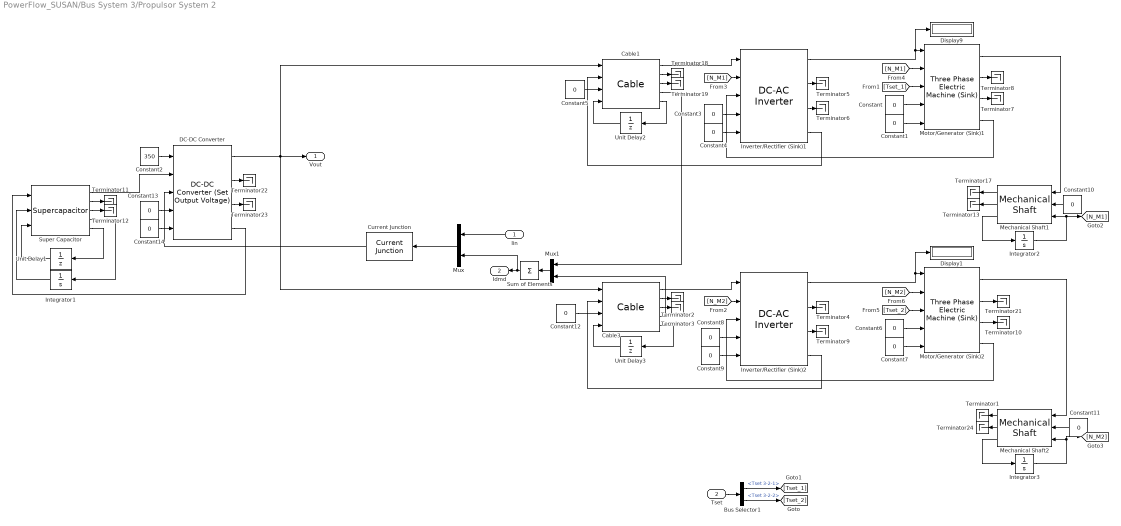
== system PowerFlow_SUSAN/Bus System 3/Propulsor System 2 ==
  Iin : Inport
  Tset : Inport  Port=2
  Bus Selector1 : BusSelector  OutputSignals=Tset 3-2-1,Tset 3-2-2
  Cable1 : Lib_EMTAT/Components/Power Flow/Cable  R=0.2
      settings: SourceProductName=EMTAT
  Cable3 : Lib_EMTAT/Components/Power Flow/Cable  R=0.2
      settings: SourceProductName=EMTAT
  Constant{,1,3..14} (14 alike) : Constant  Value=0
  Constant2 : Constant  Value=350
  Current Junction : Lib_EMTAT/Components/Power Flow/Current Junction  Nb=1
      settings: SourceProductName=EMTAT
      settings: AttributesFormatString=|
      | Current Junction
      | Version: %<LibraryVersion>
  DC-DC Converter : Lib_EMTAT/Components/Power Flow/DC-DC Converter (Set Output Voltage)  X_Vin_VoltageVec_M=[0 100 1000 5000]  Y_Iout_CurrentVec_M=[0 10 100 150]  T_C_PlossArray_M=0.98*ones(4,4)  FM=0  Plosslim=0
      settings: SourceProductName=EMTAT
  Display1 : Display
  Display9 : Display
  Integrator1 : Integrator  InitialCondition=150
  Integrator2 : Integrator  InitialCondition=2000
  Integrator3 : Integrator  InitialCondition=2000
  Inverter/Rectifier (Sink)1 : Lib_EMTAT/Components/Power Flow/DC-AC Inverter  X_C_VoltageInVec_M=[0 400]  Y_C_RMSCurrentOutVec_M=[0 300]  T_C_PowLossArray_M=[1000 1000;1000 1000]  K_e=0.0503  FM=0  Plosslim=0
      settings: SourceProductName=EMTAT
  Inverter/Rectifier (Sink)2 : Lib_EMTAT/Components/Power Flow/DC-AC Inverter  X_C_VoltageInVec_M=[0 400]  Y_C_RMSCurrentOutVec_M=[0 300]  T_C_PowLossArray_M=[1000 1000;1000 1000]  K_e=0.0503  FM=0  Plosslim=0
      settings: SourceProductName=EMTAT
  Mechanical Shaft1 : Lib_EMTAT/Components/Power Flow/Mechanical Shaft  J=0.01  B=0.001
      settings: SourceProductName=EMTAT
  Mechanical Shaft2 : Lib_EMTAT/Components/Power Flow/Mechanical Shaft  J=0.01  B=0.001
      settings: SourceProductName=EMTAT
  Motor/Generator (Sink)1 : Lib_EMTAT/Components/Power Flow/Three Phase Electric Machine (Sink)  X_C_SpeedVec_M=[0 100 1000 5000]  Y_C_TorqueVec_M=[0 10 100 150]  T_C_EffArray_M=0.99*ones(4,4)  FM=0
      settings: SourceProductName=EMTAT
  Motor/Generator (Sink)2 : Lib_EMTAT/Components/Power Flow/Three Phase Electric Machine (Sink)  X_C_SpeedVec_M=[0 100 1000 5000]  Y_C_TorqueVec_M=[0 10 100 150]  T_C_EffArray_M=0.99*ones(4,4)  FM=0
      settings: SourceProductName=EMTAT
  Mux : Mux  Inputs=2
  Mux1 : Mux  Inputs=2
  Sum of Elements : Sum  Inputs=+
  Super Capacitor : Lib_EMTAT/Components/Power Flow/Supercapacitor  C=130  ESR=0.02  TSE=0  BlkNm=double(gcb)
      settings: SourceProductName=EMTAT
  Terminator{1..13,17..19,21..24} (20 alike) : Terminator
  Unit Delay1 : UnitDelay  SampleTime=-1  HasFrameUpgradeWarning=on
  Unit Delay2 : UnitDelay  SampleTime=-1  HasFrameUpgradeWarning=on
  Unit Delay3 : UnitDelay  SampleTime=-1  HasFrameUpgradeWarning=on
  Vout : Outport
  Idmd : Outport  Port=2
  wires:
  Constant14/1 -> DC-DC Converter/5
  Constant13/1 -> DC-DC Converter/4
  Constant12/1 -> Cable3/3
  Mechanical Shaft2/2 -> Terminator24/1
  Mechanical Shaft2/1 -> Terminator1/1
  Constant11/1 -> Mechanical Shaft2/2
  Constant10/1 -> Mechanical Shaft1/2
  Mechanical Shaft1/3 -> Integrator2/1
  Motor/Generator (Sink)2/3 -> Terminator10/1
  Constant8/1 -> Inverter/Rectifier (Sink)2/4
  Inverter/Rectifier (Sink)2/1 -> Display1/1, Motor/Generator (Sink)2/1
  [N_M2] -> Motor/Generator (Sink)2/2
  Cable3/1 -> Inverter/Rectifier (Sink)2/1
  Motor/Generator (Sink)2/4 -> Inverter/Rectifier (Sink)2/3
  Constant6/1 -> Motor/Generator (Sink)2/4
  Inverter/Rectifier (Sink)2/4 -> Cable3/2
  [Tset_2] -> Motor/Generator (Sink)2/3
  Inverter/Rectifier (Sink)2/3 -> Terminator9/1
  [N_M2] -> Inverter/Rectifier (Sink)2/2
  Constant7/1 -> Motor/Generator (Sink)2/5
  Inverter/Rectifier (Sink)2/2 -> Terminator4/1
  Constant9/1 -> Inverter/Rectifier (Sink)2/5
  Constant5/1 -> Cable1/3
  Constant4/1 -> Inverter/Rectifier (Sink)1/5
  Constant3/1 -> Inverter/Rectifier (Sink)1/4
  Motor/Generator (Sink)1/3 -> Terminator7/1
  Constant1/1 -> Motor/Generator (Sink)1/5
  Constant/1 -> Motor/Generator (Sink)1/4
  Tset/1 -> Bus Selector1/1
  Bus Selector1/2 -> [Tset_2]  "<Tset 3-2-2>"
  Bus Selector1/1 -> [Tset_1]  "<Tset 3-2-1>"
  Sum of Elements/1 -> Idmd/1, Mux/2
  Mux1/1 -> Sum of Elements/1
  Motor/Generator (Sink)1/1 -> Mechanical Shaft1/1
  Inverter/Rectifier (Sink)1/2 -> Terminator5/1
  DC-DC Converter/3 -> Terminator23/1
  DC-DC Converter/2 -> Terminator22/1
  Mechanical Shaft1/1 -> Terminator17/1
  Motor/Generator (Sink)2/2 -> Terminator21/1
  Super Capacitor/3 -> Terminator12/1
  Cable1/2 -> Terminator18/1
  Motor/Generator (Sink)2/1 -> Mechanical Shaft2/1
  Cable3/3 -> Terminator3/1
  Motor/Generator (Sink)1/2 -> Terminator8/1
  Constant2/1 -> DC-DC Converter/1
  Cable1/4 -> Mux1/1
  Unit Delay1/1 -> Super Capacitor/3
  Super Capacitor/5 -> Unit Delay1/1
  Inverter/Rectifier (Sink)1/3 -> Terminator6/1
  Cable1/5 -> Unit Delay2/1
  Integrator1/1 -> Super Capacitor/2
  Inverter/Rectifier (Sink)1/4 -> Cable1/2
  Unit Delay3/1 -> Cable3/4
  Cable1/3 -> Terminator19/1
  Integrator3/1 -> Mechanical Shaft2/3, [N_M2]
  Cable3/4 -> Mux1/2
  Super Capacitor/2 -> Terminator11/1
  Inverter/Rectifier (Sink)1/1 -> Display9/1, Motor/Generator (Sink)1/1
  Cable3/5 -> Unit Delay3/1
  [N_M1] -> Inverter/Rectifier (Sink)1/2
  Cable1/1 -> Inverter/Rectifier (Sink)1/1
  Integrator2/1 -> Mechanical Shaft1/3, [N_M1]
  Mux/1 -> Current Junction/1
  Current Junction/1 -> DC-DC Converter/3
  DC-DC Converter/4 -> Super Capacitor/1
  Cable3/2 -> Terminator2/1
  Unit Delay2/1 -> Cable1/4
  Mechanical Shaft1/2 -> Terminator13/1
  [N_M1] -> Motor/Generator (Sink)1/2
  Super Capacitor/1 -> DC-DC Converter/2
  Super Capacitor/4 -> Integrator1/1
  Motor/Generator (Sink)1/4 -> Inverter/Rectifier (Sink)1/3
  DC-DC Converter/1 -> Cable1/1, Vout/1, Cable3/1
  [Tset_1] -> Motor/Generator (Sink)1/3
  Mechanical Shaft2/3 -> Integrator3/1
  Iin/1 -> Mux/1

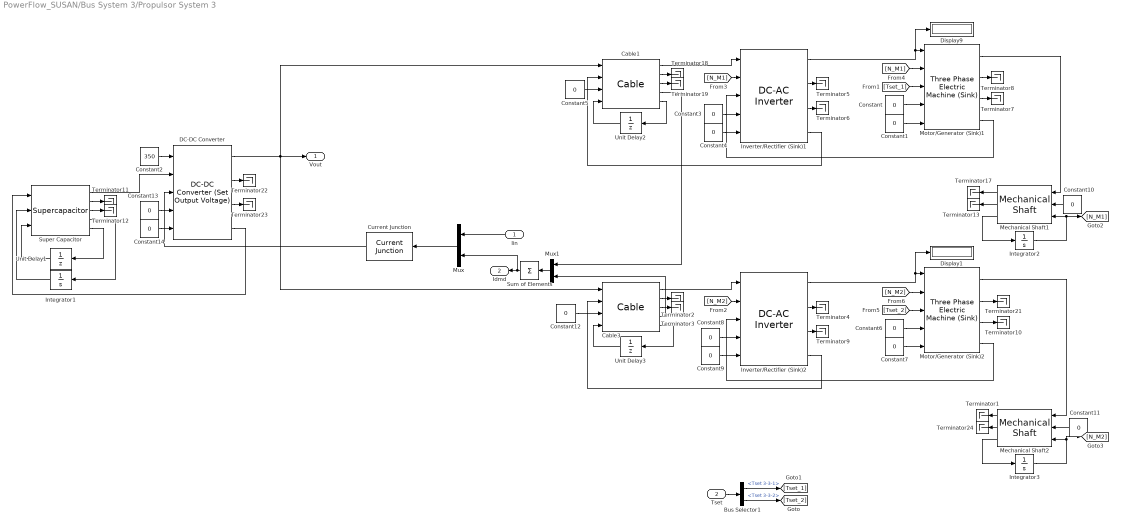
== system PowerFlow_SUSAN/Bus System 3/Propulsor System 3 ==
  Iin : Inport
  Tset : Inport  Port=2
  Bus Selector1 : BusSelector  OutputSignals=Tset 3-3-1,Tset 3-3-2
  Cable1 : Lib_EMTAT/Components/Power Flow/Cable  R=0.2
      settings: SourceProductName=EMTAT
  Cable3 : Lib_EMTAT/Components/Power Flow/Cable  R=0.2
      settings: SourceProductName=EMTAT
  Constant{,1,3..14} (14 alike) : Constant  Value=0
  Constant2 : Constant  Value=350
  Current Junction : Lib_EMTAT/Components/Power Flow/Current Junction  Nb=1
      settings: SourceProductName=EMTAT
      settings: AttributesFormatString=|
      | Current Junction
      | Version: %<LibraryVersion>
  DC-DC Converter : Lib_EMTAT/Components/Power Flow/DC-DC Converter (Set Output Voltage)  X_Vin_VoltageVec_M=[0 100 1000 5000]  Y_Iout_CurrentVec_M=[0 10 100 150]  T_C_PlossArray_M=0.98*ones(4,4)  FM=0  Plosslim=0
      settings: SourceProductName=EMTAT
  Display1 : Display
  Display9 : Display
  Integrator1 : Integrator  InitialCondition=150
  Integrator2 : Integrator  InitialCondition=2000
  Integrator3 : Integrator  InitialCondition=2000
  Inverter/Rectifier (Sink)1 : Lib_EMTAT/Components/Power Flow/DC-AC Inverter  X_C_VoltageInVec_M=[0 400]  Y_C_RMSCurrentOutVec_M=[0 300]  T_C_PowLossArray_M=[1000 1000;1000 1000]  K_e=0.0503  FM=0  Plosslim=0
      settings: SourceProductName=EMTAT
  Inverter/Rectifier (Sink)2 : Lib_EMTAT/Components/Power Flow/DC-AC Inverter  X_C_VoltageInVec_M=[0 400]  Y_C_RMSCurrentOutVec_M=[0 300]  T_C_PowLossArray_M=[1000 1000;1000 1000]  K_e=0.0503  FM=0  Plosslim=0
      settings: SourceProductName=EMTAT
  Mechanical Shaft1 : Lib_EMTAT/Components/Power Flow/Mechanical Shaft  J=0.01  B=0.001
      settings: SourceProductName=EMTAT
  Mechanical Shaft2 : Lib_EMTAT/Components/Power Flow/Mechanical Shaft  J=0.01  B=0.001
      settings: SourceProductName=EMTAT
  Motor/Generator (Sink)1 : Lib_EMTAT/Components/Power Flow/Three Phase Electric Machine (Sink)  X_C_SpeedVec_M=[0 100 1000 5000]  Y_C_TorqueVec_M=[0 10 100 150]  T_C_EffArray_M=0.99*ones(4,4)  FM=0
      settings: SourceProductName=EMTAT
  Motor/Generator (Sink)2 : Lib_EMTAT/Components/Power Flow/Three Phase Electric Machine (Sink)  X_C_SpeedVec_M=[0 100 1000 5000]  Y_C_TorqueVec_M=[0 10 100 150]  T_C_EffArray_M=0.99*ones(4,4)  FM=0
      settings: SourceProductName=EMTAT
  Mux : Mux  Inputs=2
  Mux1 : Mux  Inputs=2
  Sum of Elements : Sum  Inputs=+
  Super Capacitor : Lib_EMTAT/Components/Power Flow/Supercapacitor  C=130  ESR=0.02  TSE=0  BlkNm=double(gcb)
      settings: SourceProductName=EMTAT
  Terminator{1..13,17..19,21..24} (20 alike) : Terminator
  Unit Delay1 : UnitDelay  SampleTime=-1  HasFrameUpgradeWarning=on
  Unit Delay2 : UnitDelay  SampleTime=-1  HasFrameUpgradeWarning=on
  Unit Delay3 : UnitDelay  SampleTime=-1  HasFrameUpgradeWarning=on
  Vout : Outport
  Idmd : Outport  Port=2
  wires:
  Iin/1 -> Mux/1
  Mechanical Shaft2/3 -> Integrator3/1
  [Tset_1] -> Motor/Generator (Sink)1/3
  DC-DC Converter/1 -> Cable3/1, Vout/1, Cable1/1
  Motor/Generator (Sink)1/4 -> Inverter/Rectifier (Sink)1/3
  Super Capacitor/4 -> Integrator1/1
  Super Capacitor/1 -> DC-DC Converter/2
  [N_M1] -> Motor/Generator (Sink)1/2
  Mechanical Shaft1/2 -> Terminator13/1
  Unit Delay2/1 -> Cable1/4
  Cable3/2 -> Terminator2/1
  DC-DC Converter/4 -> Super Capacitor/1
  Current Junction/1 -> DC-DC Converter/3
  Mux/1 -> Current Junction/1
  Integrator2/1 -> [N_M1], Mechanical Shaft1/3
  Cable1/1 -> Inverter/Rectifier (Sink)1/1
  [N_M1] -> Inverter/Rectifier (Sink)1/2
  Cable3/5 -> Unit Delay3/1
  Inverter/Rectifier (Sink)1/1 -> Motor/Generator (Sink)1/1, Display9/1
  Super Capacitor/2 -> Terminator11/1
  Cable3/4 -> Mux1/2
  Integrator3/1 -> [N_M2], Mechanical Shaft2/3
  Cable1/3 -> Terminator19/1
  Unit Delay3/1 -> Cable3/4
  Inverter/Rectifier (Sink)1/4 -> Cable1/2
  Integrator1/1 -> Super Capacitor/2
  Cable1/5 -> Unit Delay2/1
  Inverter/Rectifier (Sink)1/3 -> Terminator6/1
  Super Capacitor/5 -> Unit Delay1/1
  Unit Delay1/1 -> Super Capacitor/3
  Cable1/4 -> Mux1/1
  Constant2/1 -> DC-DC Converter/1
  Motor/Generator (Sink)1/2 -> Terminator8/1
  Cable3/3 -> Terminator3/1
  Motor/Generator (Sink)2/1 -> Mechanical Shaft2/1
  Cable1/2 -> Terminator18/1
  Super Capacitor/3 -> Terminator12/1
  Motor/Generator (Sink)2/2 -> Terminator21/1
  Mechanical Shaft1/1 -> Terminator17/1
  DC-DC Converter/2 -> Terminator22/1
  DC-DC Converter/3 -> Terminator23/1
  Inverter/Rectifier (Sink)1/2 -> Terminator5/1
  Motor/Generator (Sink)1/1 -> Mechanical Shaft1/1
  Mux1/1 -> Sum of Elements/1
  Sum of Elements/1 -> Mux/2, Idmd/1
  Bus Selector1/1 -> [Tset_1]  "<Tset 3-3-1>"
  Bus Selector1/2 -> [Tset_2]  "<Tset 3-3-2>"
  Tset/1 -> Bus Selector1/1
  Constant/1 -> Motor/Generator (Sink)1/4
  Constant1/1 -> Motor/Generator (Sink)1/5
  Motor/Generator (Sink)1/3 -> Terminator7/1
  Constant3/1 -> Inverter/Rectifier (Sink)1/4
  Constant4/1 -> Inverter/Rectifier (Sink)1/5
  Constant5/1 -> Cable1/3
  Constant9/1 -> Inverter/Rectifier (Sink)2/5
  Inverter/Rectifier (Sink)2/2 -> Terminator4/1
  Constant7/1 -> Motor/Generator (Sink)2/5
  [N_M2] -> Inverter/Rectifier (Sink)2/2
  Inverter/Rectifier (Sink)2/3 -> Terminator9/1
  [Tset_2] -> Motor/Generator (Sink)2/3
  Inverter/Rectifier (Sink)2/4 -> Cable3/2
  Constant6/1 -> Motor/Generator (Sink)2/4
  Motor/Generator (Sink)2/4 -> Inverter/Rectifier (Sink)2/3
  Cable3/1 -> Inverter/Rectifier (Sink)2/1
  [N_M2] -> Motor/Generator (Sink)2/2
  Inverter/Rectifier (Sink)2/1 -> Motor/Generator (Sink)2/1, Display1/1
  Constant8/1 -> Inverter/Rectifier (Sink)2/4
  Motor/Generator (Sink)2/3 -> Terminator10/1
  Mechanical Shaft1/3 -> Integrator2/1
  Constant10/1 -> Mechanical Shaft1/2
  Constant11/1 -> Mechanical Shaft2/2
  Mechanical Shaft2/1 -> Terminator1/1
  Mechanical Shaft2/2 -> Terminator24/1
  Constant12/1 -> Cable3/3
  Constant13/1 -> DC-DC Converter/4
  Constant14/1 -> DC-DC Converter/5

== system PowerFlow_SUSAN/Bus System 3/Propulsor System 4 ==
  Iin : Inport
  Tset : Inport  Port=2
  Bus Selector1 : BusSelector  OutputSignals=Tset 3-4-1,Tset 3-4-2
  Cable1 : Lib_EMTAT/Components/Power Flow/Cable  R=0.2
      settings: SourceProductName=EMTAT
  Cable3 : Lib_EMTAT/Components/Power Flow/Cable  R=0.2
      settings: SourceProductName=EMTAT
  Constant{,1,3..14} (14 alike) : Constant  Value=0
  Constant2 : Constant  Value=350
  Current Junction : Lib_EMTAT/Components/Power Flow/Current Junction  Nb=1
      settings: SourceProductName=EMTAT
      settings: AttributesFormatString=|
      | Current Junction
      | Version: %<LibraryVersion>
  DC-DC Converter : Lib_EMTAT/Components/Power Flow/DC-DC Converter (Set Output Voltage)  X_Vin_VoltageVec_M=[0 100 1000 5000]  Y_Iout_CurrentVec_M=[0 10 100 150]  T_C_PlossArray_M=0.98*ones(4,4)  FM=0  Plosslim=0
      settings: SourceProductName=EMTAT
  Display1 : Display
  Display9 : Display
  Integrator1 : Integrator  InitialCondition=150
  Integrator2 : Integrator  InitialCondition=2000
  Integrator3 : Integrator  InitialCondition=2000
  Inverter/Rectifier (Sink)1 : Lib_EMTAT/Components/Power Flow/DC-AC Inverter  X_C_VoltageInVec_M=[0 400]  Y_C_RMSCurrentOutVec_M=[0 300]  T_C_PowLossArray_M=[1000 1000;1000 1000]  K_e=0.0503  FM=0  Plosslim=0
      settings: SourceProductName=EMTAT
  Inverter/Rectifier (Sink)2 : Lib_EMTAT/Components/Power Flow/DC-AC Inverter  X_C_VoltageInVec_M=[0 400]  Y_C_RMSCurrentOutVec_M=[0 300]  T_C_PowLossArray_M=[1000 1000;1000 1000]  K_e=0.0503  FM=0  Plosslim=0
      settings: SourceProductName=EMTAT
  Mechanical Shaft1 : Lib_EMTAT/Components/Power Flow/Mechanical Shaft  J=0.01  B=0.001
      settings: SourceProductName=EMTAT
  Mechanical Shaft2 : Lib_EMTAT/Components/Power Flow/Mechanical Shaft  J=0.01  B=0.001
      settings: SourceProductName=EMTAT
  Motor/Generator (Sink)1 : Lib_EMTAT/Components/Power Flow/Three Phase Electric Machine (Sink)  X_C_SpeedVec_M=[0 100 1000 5000]  Y_C_TorqueVec_M=[0 10 100 150]  T_C_EffArray_M=0.99*ones(4,4)  FM=0
      settings: SourceProductName=EMTAT
  Motor/Generator (Sink)2 : Lib_EMTAT/Components/Power Flow/Three Phase Electric Machine (Sink)  X_C_SpeedVec_M=[0 100 1000 5000]  Y_C_TorqueVec_M=[0 10 100 150]  T_C_EffArray_M=0.99*ones(4,4)  FM=0
      settings: SourceProductName=EMTAT
  Mux : Mux  Inputs=2
  Mux1 : Mux  Inputs=2
  Sum of Elements : Sum  Inputs=+
  Super Capacitor : Lib_EMTAT/Components/Power Flow/Supercapacitor  C=130  ESR=0.02  TSE=0  BlkNm=double(gcb)
      settings: SourceProductName=EMTAT
  Terminator{1..13,17..19,21..24} (20 alike) : Terminator
  Unit Delay1 : UnitDelay  SampleTime=-1  HasFrameUpgradeWarning=on
  Unit Delay2 : UnitDelay  SampleTime=-1  HasFrameUpgradeWarning=on
  Unit Delay3 : UnitDelay  SampleTime=-1  HasFrameUpgradeWarning=on
  Vout : Outport
  Idmd : Outport  Port=2
  wires:
  Constant14/1 -> DC-DC Converter/5
  Constant13/1 -> DC-DC Converter/4
  Constant12/1 -> Cable3/3
  Mechanical Shaft2/2 -> Terminator24/1
  Mechanical Shaft2/1 -> Terminator1/1
  Constant11/1 -> Mechanical Shaft2/2
  Constant10/1 -> Mechanical Shaft1/2
  Mechanical Shaft1/3 -> Integrator2/1
  Motor/Generator (Sink)2/3 -> Terminator10/1
  Constant8/1 -> Inverter/Rectifier (Sink)2/4
  Inverter/Rectifier (Sink)2/1 -> Display1/1, Motor/Generator (Sink)2/1
  [N_M2] -> Motor/Generator (Sink)2/2
  Cable3/1 -> Inverter/Rectifier (Sink)2/1
  Motor/Generator (Sink)2/4 -> Inverter/Rectifier (Sink)2/3
  Constant6/1 -> Motor/Generator (Sink)2/4
  Inverter/Rectifier (Sink)2/4 -> Cable3/2
  [Tset_2] -> Motor/Generator (Sink)2/3
  Inverter/Rectifier (Sink)2/3 -> Terminator9/1
  [N_M2] -> Inverter/Rectifier (Sink)2/2
  Constant7/1 -> Motor/Generator (Sink)2/5
  Inverter/Rectifier (Sink)2/2 -> Terminator4/1
  Constant9/1 -> Inverter/Rectifier (Sink)2/5
  Constant5/1 -> Cable1/3
  Constant4/1 -> Inverter/Rectifier (Sink)1/5
  Constant3/1 -> Inverter/Rectifier (Sink)1/4
  Motor/Generator (Sink)1/3 -> Terminator7/1
  Constant1/1 -> Motor/Generator (Sink)1/5
  Constant/1 -> Motor/Generator (Sink)1/4
  Tset/1 -> Bus Selector1/1
  Bus Selector1/2 -> [Tset_2]  "<Tset 3-4-2>"
  Bus Selector1/1 -> [Tset_1]  "<Tset 3-4-1>"
  Sum of Elements/1 -> Idmd/1, Mux/2
  Mux1/1 -> Sum of Elements/1
  Motor/Generator (Sink)1/1 -> Mechanical Shaft1/1
  Inverter/Rectifier (Sink)1/2 -> Terminator5/1
  DC-DC Converter/3 -> Terminator23/1
  DC-DC Converter/2 -> Terminator22/1
  Mechanical Shaft1/1 -> Terminator17/1
  Motor/Generator (Sink)2/2 -> Terminator21/1
  Super Capacitor/3 -> Terminator12/1
  Cable1/2 -> Terminator18/1
  Motor/Generator (Sink)2/1 -> Mechanical Shaft2/1
  Cable3/3 -> Terminator3/1
  Motor/Generator (Sink)1/2 -> Terminator8/1
  Constant2/1 -> DC-DC Converter/1
  Cable1/4 -> Mux1/1
  Unit Delay1/1 -> Super Capacitor/3
  Super Capacitor/5 -> Unit Delay1/1
  Inverter/Rectifier (Sink)1/3 -> Terminator6/1
  Cable1/5 -> Unit Delay2/1
  Integrator1/1 -> Super Capacitor/2
  Inverter/Rectifier (Sink)1/4 -> Cable1/2
  Unit Delay3/1 -> Cable3/4
  Cable1/3 -> Terminator19/1
  Integrator3/1 -> Mechanical Shaft2/3, [N_M2]
  Cable3/4 -> Mux1/2
  Super Capacitor/2 -> Terminator11/1
  Inverter/Rectifier (Sink)1/1 -> Display9/1, Motor/Generator (Sink)1/1
  Cable3/5 -> Unit Delay3/1
  [N_M1] -> Inverter/Rectifier (Sink)1/2
  Cable1/1 -> Inverter/Rectifier (Sink)1/1
  Integrator2/1 -> Mechanical Shaft1/3, [N_M1]
  Mux/1 -> Current Junction/1
  Current Junction/1 -> DC-DC Converter/3
  DC-DC Converter/4 -> Super Capacitor/1
  Cable3/2 -> Terminator2/1
  Unit Delay2/1 -> Cable1/4
  Mechanical Shaft1/2 -> Terminator13/1
  [N_M1] -> Motor/Generator (Sink)1/2
  Super Capacitor/1 -> DC-DC Converter/2
  Super Capacitor/4 -> Integrator1/1
  Motor/Generator (Sink)1/4 -> Inverter/Rectifier (Sink)1/3
  DC-DC Converter/1 -> Cable1/1, Vout/1, Cable3/1
  [Tset_1] -> Motor/Generator (Sink)1/3
  Mechanical Shaft2/3 -> Integrator3/1
  Iin/1 -> Mux/1
